simulink model "PIDPrax"  (R2018a)
settings: Solver=VariableStepAuto  StartTime=0.0  StopTime=10  RelTol=1e-3
libraries: simulink x1
settings Model: Creator=ACALVILLM  LastModifiedBy=ACALVILLM

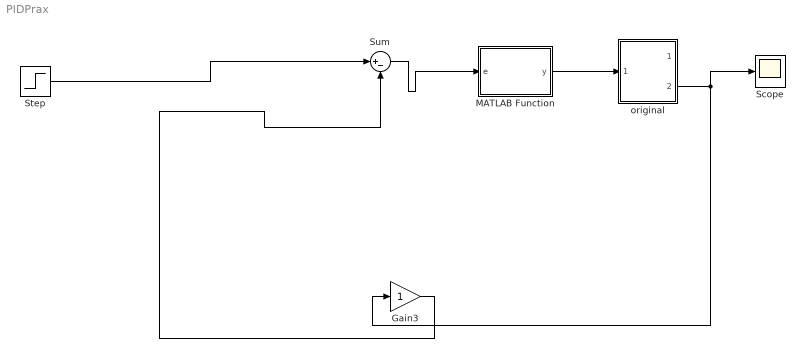
== system PIDPrax ==
  Gain3 : Gain
  MATLAB Function : MATLAB Function  TreatAsAtomicUnit=on
  Scope : Scope
  Step : Step  After=4  SampleTime=1
  Sum : Sum  Inputs=|+-
  original : Subsystem
  wires:
  original/2(clean) -> Gain3/1, Scope/1
  MATLAB Function/1(y) -> original/1("MotoMoto ")
  Sum/1 -> MATLAB Function/1(e)
  Gain3/1 -> Sum/2
  Step/1 -> Sum/1

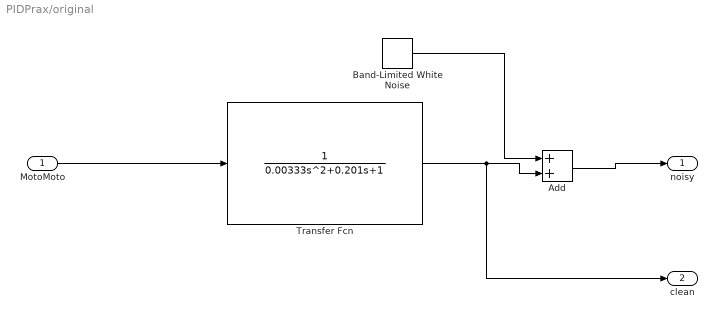
== system PIDPrax/original ==
  "MotoMoto " : Inport
  Add : Sum
  Band-Limited White Noise : simulink/Sources/Band-Limited White Noise  Cov=[0.0000001]  Ts=0.001  seed=[23341]
  Transfer Fcn : TransferFcn  Denominator=[0.00333 0.201 1]
  noisy : Outport
  clean : Outport  Port=2
  wires:
  Transfer Fcn/1 -> clean/1, Add/2
  Band-Limited White Noise/1 -> Add/1
  Add/1 -> noisy/1
  "MotoMoto "/1 -> Transfer Fcn/1

== matlab function PIDPrax/MATLAB Function ==
  data: e input; y output

function y = PID(e)
coder.extrinsic('evalin');
coder.extrinsic('assignin');
e0=0;
err=0;
ki=0.0113;
kp=58.8235;
kd=22.6/8000;
%PID
e0=evalin('base','e0');
err=evalin('base','error');
integ=err+e;
di=(e-e0);
assignin('caller','t0',t1);
assignin('caller','e0',e);
assignin('caller','error',integ);
u=kp*e+ki*integ+kd*di;
y = u;
end
